simulink model "MBDMotorSystemUpd1MaxIaLmt"  (R2023a)
settings: Solver=VariableStepAuto  StartTime=0.0  StopTime=0.5  RelTol=1e-3
undefined symbols (not defined in the file or in its folder): CntFdqDcpMap, CntLdqDMap, CntTrqReqMap, DiscIntNeverNeededParam, Izc, Izr, MdlFluxMap, MdlTrqMap, Pos0
libraries: simulink x30, simulink_extras x6
(part 4 of 4)

== system MBDMotorSystemUpd1MaxIaLmt/PM Controller/Modulator/Over Modulation/Ovr. Mod./OvrMod. SPWM ==
  Mr : Inport
  Action Port : ActionPort  ActionPortLabel=default:
  Compare To Constant : simulink/Logic and Bit Operations/Compare To Constant  relop=>  const=1/sqrt(2)  OutDataTypeStr=boolean
  Ovr SPWM : Lookup_n-D  NumberOfTableDimensions=1  BreakpointsForDimension1=[0.7, 0.7001, 0.7002, 0.7003, 0.7004, 0.7005, 0.7006, 0.7007, 0.7008, 0.7009, 0.701, 0.7011, 0.7012, 0.7013, 0.7014, 0.7015, 0.7016, 0.7017, 0.7018, 0.7019, 0.702, 0.7021, 0.7022, 0.7023, 0.7024, 0.7025, 0.7026, 0.7027, 0.7028, 0.7029, 0.703, 0.7031, 0.7032, 0.7033, 0.7034, 0.7035, 0.7036, 0.7037, 0.7038, 0.7039, 0.704, 0.7041, 0.7042, 0.7043, 0.7044, 0.7045, 0.7046, 0.7047, 0.7048, 0.7049, 0.705, 0.7051, 0.7052, 0.7053, 0.7054, 0.7055, 0.7056, 0.7057, 0.7058, 0.7059, 0.706, 0.7061, 0.7062, 0.7063, 0.7064, 0.7065, 0.7066, 0.7067, 0.7068, 0.7069, 0.707, 0.7071, 0.7072, 0.7073, 0.7074, 0.7075, 0.7076, 0.7077, 0.7078, 0.7079, 0.708, 0.7081, 0.7082, 0.7083, 0.7084, 0.7085, 0.7086, 0.7087, 0.7088, 0.7089, 0.709, 0.7091, 0.7092, 0.7093, 0.7094, 0.7095, 0.7096, 0.7097, 0.7098, 0.7099, 0.71, 0.7101, 0.7102, 0.7103, 0.7104, 0.7105, 0.7106, 0.7107, 0.7108, 0.7109, 0.711, 0.7111, 0.7112, 0.7113, 0.7114, 0.7115, 0.7116, 0.7117, 0.7118, 0.7119, 0.712, 0.7121, 0.7122, 0.7123, 0.7124, 0.7125, 0.7126, 0.7127, 0.7128, 0.7129, 0.713, 0.7131, 0.7132, 0.7133, 0.7134, 0.7135, 0.7136, 0.7137, 0.7138, 0.7139, 0.714, 0.7141, 0.7142, 0.7143, 0.7144, 0.7145, 0.7146, 0.7147, 0.7148, 0.7149, 0.715, 0.7151, 0.7152, 0.7153, 0.7154, 0.7155, 0.7156, 0.7157, 0.7158, 0.7159, 0.716, 0.7161, 0.7162, 0.7163, 0.7164, 0.7165, 0.7166, 0.7167, 0.7168, 0.7169, 0.717, 0.7171, 0.7172, 0.7173, 0.7174, 0.7175, 0.7176, 0.7177, 0.7178, 0.7179, 0.718, 0.7181, 0.7182, 0.7183, 0.7184, 0.7185, 0.7186, 0.7187, 0.7188, 0.7189, 0.719, 0.7191, 0.7192, 0.7193, 0.7194, 0.7195, 0.7196, 0.7197, 0.7198, 0.7199, 0.72, 0.7201, 0.7202, 0.7203, 0.7204, 0.7205, 0.7206, 0.7207, 0.7208, 0.7209, 0.721, 0.7211, 0.7212, 0.7213, 0.7214, 0.7215, 0.7216, 0.7217, 0.7218, 0.7219, 0.722, 0.7221, 0.7222, 0.7223, 0.7224, 0.7225, 0.7226, 0.7227, 0.7228, 0.7229, 0.723, 0.7231, 0.7232, 0.7233, 0.7234, 0.7235, 0.7236, 0.7237, 0.7238, 0.7239, 0.724, 0.7241, 0.7242, 0.7243, 0.7244, 0.7245, 0.7246, 0.7247, 0.7248, 0.7249, 0.725, 0.7251, 0.7252, 0.7253, 0.7254, 0.7255, 0.7256, 0.7257, 0.7258, 0.7259, 0.726, 0.7261, 0.7262, 0.7263, 0.7264, 0.7265, 0.7266, 0.7267, 0.7268, 0.7269, 0.727, 0.7271, 0.7272, 0.7273, 0.7274, 0.7275, 0.7276, 0.7277, 0.7278, 0.7279, 0.728, 0.7281, 0.7282, 0.7283, 0.7284, 0.7285, 0.7286, 0.7287, 0.7288, 0.7289, 0.729, 0.7291, 0.7292, 0.7293, 0.7294, 0.7295, 0.7296, 0.7297, 0.7298, 0.7299, 0.73, 0.7301, 0.7302, 0.7303, 0.7304, 0.7305, 0.7306, 0.7307, 0.7308, 0.7309, 0.731, 0.7311, 0.7312, 0.7313, 0.7314, 0.7315, 0.7316, 0.7317, 0.7318, 0.7319, 0.732, 0.7321, 0.7322, 0.7323, 0.7324, 0.7325, 0.7326, 0.7327, 0.7328, 0.7329, 0.733, 0.7331, 0.7332, 0.7333, 0.7334, 0.7335, 0.7336, 0.7337, 0.7338, 0.7339, 0.734, 0.7341, 0.7342, 0.7343, 0.7344, 0.7345, 0.7346, 0.7347, 0.7348, 0.7349, 0.735, 0.7351, 0.7352, 0.7353, 0.7354, 0.7355, 0.7356, 0.7357, 0.7358, 0.7359, 0.736, 0.7361, 0.7362, 0.7363, 0.7364, 0.7365, 0.7366, 0.7367, 0.7368, 0.7369, 0.737, 0.7371, 0.7372, 0.7373, 0.7374, 0.7375, 0.7376, 0.7377, 0.7378, 0.7379, 0.738, 0.7381, 0.7382, 0.7383, 0.7384, 0.7385, 0.7386, 0.7387, 0.7388, 0.7389, 0.739, 0.7391, 0.7392, 0.7393, 0.7394, 0.7395, 0.7396, 0.7397, 0.7398, 0.7399, 0.74, 0.7401, 0.7402, 0.7403, 0.7404, 0.7405, 0.7406, 0.7407, 0.7408, 0.7409, 0.741, 0.7411, 0.7412, 0.7413, 0.7414, 0.7415, 0.7416, 0.7417, 0.7418, 0.7419, 0.742, 0.7421, 0.7422, 0.7423, 0.7424, 0.7425, 0.7426, 0.7427, 0.7428, 0.7429, 0.743, 0.7431, 0.7432, 0.7433, 0.7434, 0.7435, 0.7436, 0.7437, 0.7438, 0.7439, 0.744, 0.7441, 0.7442, 0.7443, 0.7444, 0.7445, 0.7446, 0.7447, 0.7448, 0.7449, 0.745, 0.7451, 0.7452, 0.7453, 0.7454, 0.7455, 0.7456, 0.7457, 0.7458, 0.7459, 0.746, 0.7461, 0.7462, 0.7463, 0.7464, 0.7465, 0.7466, 0.7467, 0.7468, 0.7469, 0.747, 0.7471, 0.7472, 0.7473, 0.7474, 0.7475, 0.7476, 0.7477, 0.7478, 0.7479, 0.748, 0.7481, 0.7482, 0.7483, 0.7484, 0.7485, 0.7486, 0.7487, 0.7488, 0.7489, 0.749, 0.7491, 0.7492, 0.7493, 0.7494, 0.7495, 0.7496, 0.7497, 0.7498, 0.7499, 0.75, 0.7501, 0.7502, 0.7503, 0.7504, 0.7505, 0.7506, ...(+2240 chars)]  IndexSearchMethod=Evenly spaced points  Table=[0.822459, 0.822918, 0.823377, 0.823838, 0.824299, 0.824762, 0.825225, 0.825689, 0.826154, 0.82662, 0.827087, 0.827555, 0.828024, 0.828494, 0.828965, 0.829437, 0.82991, 0.830383, 0.830858, 0.831334, 0.831811, 0.832288, 0.832767, 0.833247, 0.833727, 0.834209, 0.834691, 0.835175, 0.83566, 0.836145, 0.836632, 0.837119, 0.837608, 0.838098, 0.838588, 0.83908, 0.839573, 0.840067, 0.840562, 0.841057, 0.841554, 0.842052, 0.842551, 0.843051, 0.843552, 0.844055, 0.844558, 0.845062, 0.845567, 0.846074, 0.846581, 0.84709, 0.8476, 0.84811, 0.848622, 0.849135, 0.849649, 0.850164, 0.850681, 0.851198, 0.851717, 0.852236, 0.852757, 0.853279, 0.853802, 0.854326, 0.854851, 0.855378, 0.855905, 0.856434, 0.856964, 0.857495, 0.858027, 0.85856, 0.859095, 0.85963, 0.860167, 0.860705, 0.861244, 0.861785, 0.862326, 0.862869, 0.863413, 0.863958, 0.864505, 0.865052, 0.865601, 0.866151, 0.866702, 0.867255, 0.867809, 0.868364, 0.86892, 0.869477, 0.870036, 0.870596, 0.871157, 0.87172, 0.872284, 0.872849, 0.873415, 0.873983, 0.874552, 0.875122, 0.875693, 0.876266, 0.87684, 0.877416, 0.877993, 0.878571, 0.87915, 0.879731, 0.880313, 0.880896, 0.881481, 0.882067, 0.882654, 0.883243, 0.883833, 0.884425, 0.885018, 0.885612, 0.886208, 0.886805, 0.887404, 0.888003, 0.888605, 0.889207, 0.889812, 0.890417, 0.891024, 0.891632, 0.892242, 0.892854, 0.893466, 0.894081, 0.894696, 0.895313, 0.895932, 0.896552, 0.897174, 0.897797, 0.898421, 0.899047, 0.899675, 0.900304, 0.900934, 0.901566, 0.9022, 0.902835, 0.903472, 0.90411, 0.90475, 0.905391, 0.906034, 0.906679, 0.907325, 0.907972, 0.908621, 0.909272, 0.909925, 0.910579, 0.911234, 0.911892, 0.91255, 0.913211, 0.913873, 0.914537, 0.915202, 0.91587, 0.916538, 0.917209, 0.917881, 0.918555, 0.91923, 0.919907, 0.920586, 0.921267, 0.921949, 0.922633, 0.923319, 0.924007, 0.924696, 0.925387, 0.92608, 0.926774, 0.927471, 0.928169, 0.928869, 0.929571, 0.930274, 0.93098, 0.931687, 0.932396, 0.933107, 0.933819, 0.934534, 0.93525, 0.935968, 0.936688, 0.93741, 0.938134, 0.93886, 0.939588, 0.940317, 0.941049, 0.941782, 0.942518, 0.943255, 0.943995, 0.944736, 0.945479, 0.946224, 0.946971, 0.947721, 0.948472, 0.949225, 0.94998, 0.950738, 0.951497, 0.952258, 0.953022, 0.953787, 0.954555, 0.955324, 0.956096, 0.95687, 0.957646, 0.958424, 0.959204, 0.959986, 0.960771, 0.961558, 0.962346, 0.963137, 0.963931, 0.964726, 0.965524, 0.966323, 0.967125, 0.96793, 0.968736, 0.969545, 0.970356, 0.971169, 0.971985, 0.972803, 0.973623, 0.974446, 0.97527, 0.976098, 0.976927, 0.977759, 0.978593, 0.97943, 0.980269, 0.981111, 0.981955, 0.982801, 0.98365, 0.984501, 0.985355, 0.986211, 0.987069, 0.98793, 0.988794, 0.98966, 0.990529, 0.9914, 0.992274, 0.99315, 0.994029, 0.994911, 0.995795, 0.996682, 0.997571, 0.998463, 0.999358, 1.00026, 1.00116, 1.00206, 1.00296, 1.00387, 1.00478, 1.0057, 1.00661, 1.00753, 1.00845, 1.00938, 1.01031, 1.01124, 1.01217, 1.01311, 1.01404, 1.01499, 1.01593, 1.01688, 1.01783, 1.01878, 1.01974, 1.0207, 1.02166, 1.02263, 1.0236, 1.02457, 1.02554, 1.02652, 1.0275, 1.02848, 1.02947, 1.03046, 1.03145, 1.03245, 1.03345, 1.03445, 1.03546, 1.03647, 1.03748, 1.0385, 1.03951, 1.04054, 1.04156, 1.04259, 1.04362, 1.04466, 1.0457, 1.04674, 1.04779, 1.04884, 1.04989, 1.05094, 1.052, 1.05307, 1.05413, 1.0552, 1.05628, 1.05736, 1.05844, 1.05952, 1.06061, 1.0617, 1.0628, 1.0639, 1.065, 1.06611, 1.06722, 1.06833, 1.06945, 1.07057, 1.0717, 1.07283, 1.07396, 1.0751, 1.07624, 1.07738, 1.07853, 1.07969, 1.08084, 1.08201, 1.08317, 1.08434, 1.08552, 1.08669, 1.08788, 1.08906, 1.09025, 1.09145, 1.09265, 1.09385, 1.09506, 1.09627, 1.09749, 1.09871, 1.09993, 1.10116, 1.10239, 1.10363, 1.10488, 1.10612, 1.10738, 1.10863, 1.10989, 1.11116, 1.11243, 1.11371, 1.11499, 1.11627, 1.11756, 1.11886, 1.12016, 1.12146, 1.12277, 1.12409, 1.1254, 1.12673, 1.12806, 1.12939, 1.13073, 1.13208, 1.13343, 1.13478, 1.13614, 1.13751, 1.13888, 1.14026, 1.14164, 1.14303, 1.14442, 1.14582, 1.14722, 1.14863, 1.15004, 1.15146, 1.15289, 1.15432, 1.15576, 1.1572, 1.15865, 1.16011, ...(+3309 chars)]  ExtrapMethod=Clip  UseLastTableValue=on  ApplyFullPrecisionForLinearInterpolation=on  InternalRulePriority=Speed  RndMeth=Simplest
  Switch : Switch  Criteria=u2 > Threshold  SaturateOnIntegerOverflow=off  InputSameDT=off
  Mr* : Outport
  wires:
  Switch/1 -> Mr*/1
  Mr/1 -> Switch/3, Compare To Constant/1, Ovr SPWM/1  "Normal"
  Compare To Constant/1 -> Switch/2
  Ovr SPWM/1 -> Switch/1

== system MBDMotorSystemUpd1MaxIaLmt/PM Controller/Modulator/Over Modulation/Ovr. Mod./OvrMod. SVM ==
  Mr : Inport
  Action Port : ActionPort  ActionPortLabel=case [ 0 ]:
  Compare To Constant : simulink/Logic and Bit Operations/Compare To Constant  relop=>  const=1/sqrt(2)  OutDataTypeStr=boolean
  Ovr SVM : Lookup_n-D  NumberOfTableDimensions=1  BreakpointsForDimension1=[0.7, 0.7001, 0.7002, 0.7003, 0.7004, 0.7005, 0.7006, 0.7007, 0.7008, 0.7009, 0.701, 0.7011, 0.7012, 0.7013, 0.7014, 0.7015, 0.7016, 0.7017, 0.7018, 0.7019, 0.702, 0.7021, 0.7022, 0.7023, 0.7024, 0.7025, 0.7026, 0.7027, 0.7028, 0.7029, 0.703, 0.7031, 0.7032, 0.7033, 0.7034, 0.7035, 0.7036, 0.7037, 0.7038, 0.7039, 0.704, 0.7041, 0.7042, 0.7043, 0.7044, 0.7045, 0.7046, 0.7047, 0.7048, 0.7049, 0.705, 0.7051, 0.7052, 0.7053, 0.7054, 0.7055, 0.7056, 0.7057, 0.7058, 0.7059, 0.706, 0.7061, 0.7062, 0.7063, 0.7064, 0.7065, 0.7066, 0.7067, 0.7068, 0.7069, 0.707, 0.7071, 0.7072, 0.7073, 0.7074, 0.7075, 0.7076, 0.7077, 0.7078, 0.7079, 0.708, 0.7081, 0.7082, 0.7083, 0.7084, 0.7085, 0.7086, 0.7087, 0.7088, 0.7089, 0.709, 0.7091, 0.7092, 0.7093, 0.7094, 0.7095, 0.7096, 0.7097, 0.7098, 0.7099, 0.71, 0.7101, 0.7102, 0.7103, 0.7104, 0.7105, 0.7106, 0.7107, 0.7108, 0.7109, 0.711, 0.7111, 0.7112, 0.7113, 0.7114, 0.7115, 0.7116, 0.7117, 0.7118, 0.7119, 0.712, 0.7121, 0.7122, 0.7123, 0.7124, 0.7125, 0.7126, 0.7127, 0.7128, 0.7129, 0.713, 0.7131, 0.7132, 0.7133, 0.7134, 0.7135, 0.7136, 0.7137, 0.7138, 0.7139, 0.714, 0.7141, 0.7142, 0.7143, 0.7144, 0.7145, 0.7146, 0.7147, 0.7148, 0.7149, 0.715, 0.7151, 0.7152, 0.7153, 0.7154, 0.7155, 0.7156, 0.7157, 0.7158, 0.7159, 0.716, 0.7161, 0.7162, 0.7163, 0.7164, 0.7165, 0.7166, 0.7167, 0.7168, 0.7169, 0.717, 0.7171, 0.7172, 0.7173, 0.7174, 0.7175, 0.7176, 0.7177, 0.7178, 0.7179, 0.718, 0.7181, 0.7182, 0.7183, 0.7184, 0.7185, 0.7186, 0.7187, 0.7188, 0.7189, 0.719, 0.7191, 0.7192, 0.7193, 0.7194, 0.7195, 0.7196, 0.7197, 0.7198, 0.7199, 0.72, 0.7201, 0.7202, 0.7203, 0.7204, 0.7205, 0.7206, 0.7207, 0.7208, 0.7209, 0.721, 0.7211, 0.7212, 0.7213, 0.7214, 0.7215, 0.7216, 0.7217, 0.7218, 0.7219, 0.722, 0.7221, 0.7222, 0.7223, 0.7224, 0.7225, 0.7226, 0.7227, 0.7228, 0.7229, 0.723, 0.7231, 0.7232, 0.7233, 0.7234, 0.7235, 0.7236, 0.7237, 0.7238, 0.7239, 0.724, 0.7241, 0.7242, 0.7243, 0.7244, 0.7245, 0.7246, 0.7247, 0.7248, 0.7249, 0.725, 0.7251, 0.7252, 0.7253, 0.7254, 0.7255, 0.7256, 0.7257, 0.7258, 0.7259, 0.726, 0.7261, 0.7262, 0.7263, 0.7264, 0.7265, 0.7266, 0.7267, 0.7268, 0.7269, 0.727, 0.7271, 0.7272, 0.7273, 0.7274, 0.7275, 0.7276, 0.7277, 0.7278, 0.7279, 0.728, 0.7281, 0.7282, 0.7283, 0.7284, 0.7285, 0.7286, 0.7287, 0.7288, 0.7289, 0.729, 0.7291, 0.7292, 0.7293, 0.7294, 0.7295, 0.7296, 0.7297, 0.7298, 0.7299, 0.73, 0.7301, 0.7302, 0.7303, 0.7304, 0.7305, 0.7306, 0.7307, 0.7308, 0.7309, 0.731, 0.7311, 0.7312, 0.7313, 0.7314, 0.7315, 0.7316, 0.7317, 0.7318, 0.7319, 0.732, 0.7321, 0.7322, 0.7323, 0.7324, 0.7325, 0.7326, 0.7327, 0.7328, 0.7329, 0.733, 0.7331, 0.7332, 0.7333, 0.7334, 0.7335, 0.7336, 0.7337, 0.7338, 0.7339, 0.734, 0.7341, 0.7342, 0.7343, 0.7344, 0.7345, 0.7346, 0.7347, 0.7348, 0.7349, 0.735, 0.7351, 0.7352, 0.7353, 0.7354, 0.7355, 0.7356, 0.7357, 0.7358, 0.7359, 0.736, 0.7361, 0.7362, 0.7363, 0.7364, 0.7365, 0.7366, 0.7367, 0.7368, 0.7369, 0.737, 0.7371, 0.7372, 0.7373, 0.7374, 0.7375, 0.7376, 0.7377, 0.7378, 0.7379, 0.738, 0.7381, 0.7382, 0.7383, 0.7384, 0.7385, 0.7386, 0.7387, 0.7388, 0.7389, 0.739, 0.7391, 0.7392, 0.7393, 0.7394, 0.7395, 0.7396, 0.7397, 0.7398, 0.7399, 0.74, 0.7401, 0.7402, 0.7403, 0.7404, 0.7405, 0.7406, 0.7407, 0.7408, 0.7409, 0.741, 0.7411, 0.7412, 0.7413, 0.7414, 0.7415, 0.7416, 0.7417, 0.7418, 0.7419, 0.742, 0.7421, 0.7422, 0.7423, 0.7424, 0.7425, 0.7426, 0.7427, 0.7428, 0.7429, 0.743, 0.7431, 0.7432, 0.7433, 0.7434, 0.7435, 0.7436, 0.7437, 0.7438, 0.7439, 0.744, 0.7441, 0.7442, 0.7443, 0.7444, 0.7445, 0.7446, 0.7447, 0.7448, 0.7449, 0.745, 0.7451, 0.7452, 0.7453, 0.7454, 0.7455, 0.7456, 0.7457, 0.7458, 0.7459, 0.746, 0.7461, 0.7462, 0.7463, 0.7464, 0.7465, 0.7466, 0.7467, 0.7468, 0.7469, 0.747, 0.7471, 0.7472, 0.7473, 0.7474, 0.7475, 0.7476, 0.7477, 0.7478, 0.7479, 0.748, 0.7481, 0.7482, 0.7483, 0.7484, 0.7485, 0.7486, 0.7487, 0.7488, 0.7489, 0.749, 0.7491, 0.7492, 0.7493, 0.7494, 0.7495, 0.7496, 0.7497, 0.7498, 0.7499, 0.75, 0.7501, 0.7502, 0.7503, 0.7504, 0.7505, 0.7506, ...(+2240 chars)]  IndexSearchMethod=Evenly spaced points  Table=[0.7, 0.7001, 0.7002, 0.7003, 0.7004, 0.7005, 0.7006, 0.7007, 0.7008, 0.7009, 0.701, 0.7011, 0.7012, 0.7013, 0.7014, 0.7015, 0.7016, 0.7017, 0.7018, 0.7019, 0.702, 0.7021, 0.7022, 0.7023, 0.7024, 0.7025, 0.7026, 0.7027, 0.7028, 0.7029, 0.703, 0.7031, 0.7032, 0.7033, 0.7034, 0.7035, 0.7036, 0.7037, 0.7038, 0.7039, 0.704, 0.7041, 0.7042, 0.7043, 0.7044, 0.7045, 0.7046, 0.7047, 0.7048, 0.7049, 0.705, 0.7051, 0.7052, 0.7053, 0.7054, 0.7055, 0.7056, 0.7057, 0.7058, 0.7059, 0.706, 0.7061, 0.706199, 0.706298, 0.706397, 0.706496, 0.706596, 0.706696, 0.706796, 0.706898, 0.707, 0.707103, 0.707207, 0.707311, 0.707417, 0.707522, 0.707629, 0.707736, 0.707844, 0.707953, 0.708063, 0.708174, 0.708286, 0.708398, 0.708512, 0.708626, 0.708741, 0.708857, 0.708972, 0.709088, 0.709205, 0.709323, 0.709441, 0.709559, 0.709679, 0.709798, 0.709918, 0.710039, 0.71016, 0.710282, 0.710404, 0.710527, 0.71065, 0.710774, 0.710898, 0.711023, 0.711148, 0.711274, 0.7114, 0.711527, 0.711654, 0.711782, 0.71191, 0.712038, 0.712167, 0.712297, 0.712427, 0.712557, 0.712688, 0.71282, 0.712952, 0.713084, 0.713217, 0.71335, 0.713484, 0.713619, 0.713753, 0.713889, 0.714024, 0.71416, 0.714297, 0.714434, 0.714572, 0.71471, 0.714848, 0.714987, 0.715127, 0.715267, 0.715407, 0.715548, 0.715689, 0.715831, 0.715973, 0.716116, 0.716259, 0.716403, 0.716547, 0.716692, 0.716837, 0.716983, 0.717129, 0.717275, 0.717423, 0.71757, 0.717718, 0.717867, 0.718016, 0.718165, 0.718315, 0.718466, 0.718617, 0.718768, 0.71892, 0.719072, 0.719225, 0.719379, 0.719533, 0.719687, 0.719842, 0.719997, 0.720153, 0.72031, 0.720467, 0.720624, 0.720782, 0.720941, 0.7211, 0.721259, 0.721419, 0.72158, 0.721741, 0.721902, 0.722064, 0.722227, 0.72239, 0.722554, 0.722718, 0.722883, 0.723048, 0.723214, 0.72338, 0.723547, 0.723714, 0.723882, 0.724051, 0.72422, 0.72439, 0.72456, 0.724731, 0.724902, 0.725074, 0.725246, 0.725419, 0.725593, 0.725767, 0.725941, 0.726117, 0.726293, 0.726469, 0.726646, 0.726824, 0.727002, 0.727181, 0.72736, 0.72754, 0.72772, 0.727902, 0.728083, 0.728266, 0.728449, 0.728632, 0.728817, 0.729001, 0.729187, 0.729373, 0.72956, 0.729747, 0.729935, 0.730124, 0.730313, 0.730503, 0.730694, 0.730885, 0.731077, 0.731269, 0.731462, 0.731656, 0.731851, 0.732046, 0.732242, 0.732439, 0.732636, 0.732834, 0.733033, 0.733232, 0.733432, 0.733633, 0.733834, 0.734037, 0.73424, 0.734443, 0.734648, 0.734853, 0.735059, 0.735265, 0.735472, 0.735681, 0.735889, 0.736099, 0.736309, 0.736521, 0.736733, 0.736945, 0.737159, 0.737373, 0.737588, 0.737804, 0.738021, 0.738238, 0.738457, 0.738676, 0.738896, 0.739117, 0.739338, 0.739561, 0.739784, 0.740008, 0.740233, 0.740459, 0.740686, 0.740914, 0.741143, 0.741372, 0.741603, 0.741834, 0.742066, 0.742299, 0.742533, 0.742768, 0.743004, 0.743241, 0.743479, 0.743718, 0.743958, 0.744199, 0.744441, 0.744684, 0.744927, 0.745172, 0.745418, 0.745665, 0.745913, 0.746162, 0.746412, 0.746663, 0.746915, 0.747169, 0.747423, 0.747679, 0.747935, 0.748193, 0.748452, 0.748712, 0.748973, 0.749236, 0.749499, 0.749764, 0.75003, 0.750297, 0.750565, 0.750835, 0.751106, 0.751378, 0.751651, 0.751926, 0.752202, 0.752479, 0.752758, 0.753038, 0.753319, 0.753602, 0.753886, 0.754171, 0.754458, 0.754746, 0.755036, 0.755327, 0.755619, 0.755913, 0.756209, 0.756506, 0.756805, 0.757105, 0.757407, 0.75771, 0.758015, 0.758321, 0.75863, 0.758939, 0.759251, 0.759564, 0.759879, 0.760196, 0.760514, 0.760834, 0.761157, 0.76148, 0.761806, 0.762134, 0.762463, 0.762795, 0.763128, 0.763463, 0.763801, 0.76414, 0.764482, 0.764825, 0.765171, 0.765519, 0.765869, 0.766221, 0.766576, 0.766932, 0.767291, 0.767653, 0.768016, 0.768383, 0.768751, 0.769123, 0.769496, 0.769872, 0.770251, 0.770633, 0.771017, 0.771404, 0.771794, 0.772186, 0.772582, 0.77298, 0.773382, 0.773786, 0.774194, 0.774605, 0.775019, 0.775436, 0.775857, 0.776281, 0.776708, 0.777139, 0.777574, 0.778012, 0.778454, 0.7789, 0.77935, 0.779804, 0.780262, 0.780725, 0.781191, 0.781662, 0.782137, 0.782617, 0.783102, 0.783592, 0.784086, 0.784586, 0.785091, 0.785601 ...(+3472 chars)]  ExtrapMethod=Clip  UseLastTableValue=on  ApplyFullPrecisionForLinearInterpolation=on  InternalRulePriority=Speed  RndMeth=Simplest
  Scope : Scope  NumInputPorts=2
  Selector : Selector  InputPortWidth=3  IndexOptions=Index vector (dialog)  Indices=1  OutputSizes=1
  Selector1 : Selector  InputPortWidth=3  IndexOptions=Index vector (dialog)  Indices=1  OutputSizes=1
  Signal Conversion : SignalConversion  OverrideOpt=off
  Switch : Switch  Criteria=u2 > Threshold  SaturateOnIntegerOverflow=off  InputSameDT=off
  Mr* : Outport
  wires:
  Ovr SVM/1 -> Switch/1
  Compare To Constant/1 -> Switch/2
  Mr/1 -> Selector1/1, Ovr SVM/1, Compare To Constant/1, Switch/3  "Normal"
  Switch/1 -> Signal Conversion/1, Mr*/1
  Signal Conversion/1 -> Selector/1
  Selector1/1 -> Scope/2
  Selector/1 -> Scope/1
